simulink model "b2"  (R2020b)
settings: Solver=VariableStepAuto  StartTime=0.0  StopTime=inf  RelTol=1e-3
settings Model: Creator=Taha  LastModifiedBy=Taha

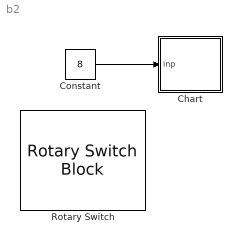
== system b2 ==
  Chart : Stateflow chart  TreatAsAtomicUnit=on
  Constant : Constant  Value=8
  Rotary Switch : RotarySwitchBlock
      settings: Values={{'b', 'a', 'c', 'd', 'e', 'f', 'g', 'h'}, [1 2 3 4 5 6 7 8]}
  wires:
  Constant/1 -> Chart/1(inp)

== stateflow chart b2/Chart ==
  state Z
    state M [parallel]
      settings: executionOrder=1
      (history)
      state Y
        (history)
        state Q
        state P
        P -> Q : [inp == 8]
        Q -> P : [inp == 7]
        (default) -> P
      state X
      (default) -> X
      X -> Y : [inp == 3]
      Y -> X : [inp == 4]
    state N [parallel]
      settings: executionOrder=2
      state S
      state R
      (default) -> R
      R -> S : [inp == 6]
      S -> R : [inp == 5]
  state T
  Z -> T : [inp == 2]
  T -> Z : [inp == 1]
  (default) -> T
  data: inp input
